simulink model "MatlabNetDDE"  (Simulink 7.3)
settings: Solver=ode3  StartTime=0.0  StopTime=inf  FixedStep=1  RelTol=1e-3
libraries: ddelib x8
settings Model: Creator=Marcin  LastModifiedBy=Marcin  ExtModeBatchMode=on  BufferReuse=off
settings DataIOCC: SaveOutput=off  SaveTime=off
settings OptimizationCC: BlockReduction=off  ConditionallyExecuteInputs=off  OptimizeBlockIOStorage=off  BufferReuse=off  ExpressionFolding=off  EnableMemcpy=off  FoldNonRolledExpr=off  LocalBlockOutputs=off  EfficientMapNaN2IntZero=off
settings RTWCC: GenerateMakefile=off  GenerateReport=on  RetainRTWFile=on  ProcessScript=grt_make_rtw_hook  LaunchReport=on  TargetLang=C++  RTWCompilerOptimization=On
settings CodeAppCC: ForceParamTrailComments=on

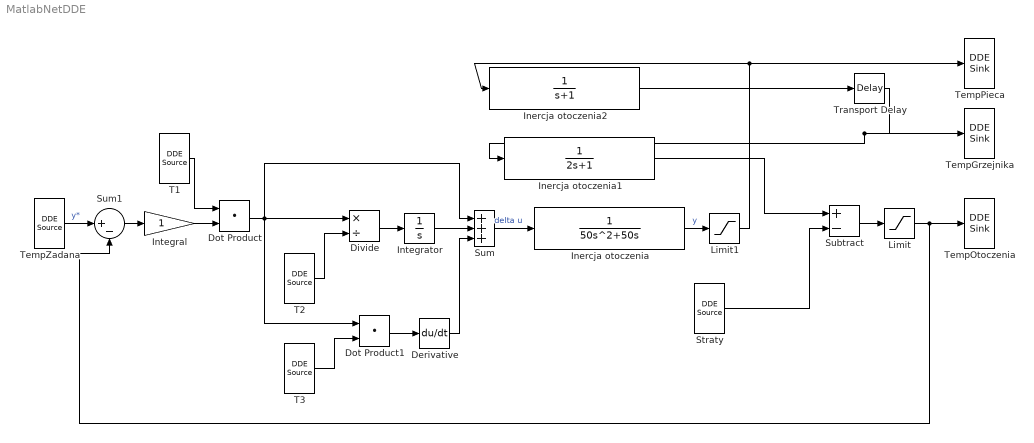
== system MatlabNetDDE ==
  Derivative : Derivative
  Divide : Product  Inputs=*/  OutDataType=fixdt(1, 16)  OutScaling=2^-10
  Dot Product : DotProduct  OutDataType=fixdt(1, 16)  OutScaling=2^-10  InputSameDT=on  OutDataTypeStr=Inherit: Inherit via internal rule
  Dot Product1 : DotProduct  OutDataType=fixdt(1, 16)  OutScaling=2^-10  InputSameDT=on  OutDataTypeStr=Inherit: Inherit via internal rule
  Inercja otoczenia : TransferFcn  Denominator=[50 50 0]
  Inercja otoczenia1 : TransferFcn  Denominator=[2 1]
  Inercja otoczenia2 : TransferFcn  Denominator=[1 1]
  Integral : Gain  ParameterDataType=sfix(16)  ParameterScaling=2^0  OutDataType=sfix(16)  OutScaling=2^0  SaturateOnIntegerOverflow=on  OutDataTypeStr=Inherit: Same as input  ParamDataTypeStr=Inherit: Same as input
  Integrator : Integrator
  Limit : Saturate  UpperLimit=100  LowerLimit=0  OutDataType=fixdt(1, 16)  OutScaling=2^0
  Limit1 : Saturate  UpperLimit=100  LowerLimit=0  OutDataType=fixdt(1, 16)  OutScaling=2^0
  Straty : ddelib/DDE Source  SystemSampleTime=-1  service='\\PC3\NDDE$'  topic='intouch$'  item='Straty'
  Subtract : Sum  Inputs=+-  OutDataType=fixdt(1, 16)  OutScaling=2^-10
  Sum : Sum  Inputs=+++  OutDataType=sfix(16)  OutScaling=2^0  SaturateOnIntegerOverflow=on  InputSameDT=on  OutDataTypeStr=Inherit: Same as first input
  Sum1 : Sum  Inputs=|+-  OutDataType=sfix(16)  OutScaling=2^0  SaturateOnIntegerOverflow=on
  T1 : ddelib/DDE Source  SystemSampleTime=-1  service='\\PC3\NDDE$'  topic='intouch$'  item='T1'
  T2 : ddelib/DDE Source  SystemSampleTime=-1  service='\\PC3\NDDE$'  topic='intouch$'  item='T2'
  T3 : ddelib/DDE Source  SystemSampleTime=-1  service='\\PC3\NDDE$'  topic='intouch$'  item='T3'
  TempGrzejnika : ddelib/DDE Sink  SystemSampleTime=-1  service='\\PC3\NDDE$'  topic='intouch$'  item='TempGrzejnika'
  TempOtoczenia : ddelib/DDE Sink  SystemSampleTime=-1  service='\\PC3\NDDE$'  topic='intouch$'  item='TempOtoczenia'
  TempPieca : ddelib/DDE Sink  SystemSampleTime=-1  service='\\PC3\NDDE$'  topic='intouch$'  item='TempPieca'
  TempZadana : ddelib/DDE Source  SystemSampleTime=-1  service='\\PC3\NDDE$'  topic='intouch$'  item='TempZadanaOtoczenia'
  Transport Delay : TransportDelay
  wires:
  Integrator/1 -> Sum/2
  Sum/1 -> Inercja otoczenia/1  "delta u"
  Divide/1 -> Integrator/1
  Dot Product1/1 -> Derivative/1
  T3/1 -> Dot Product1/2
  T1/1 -> Dot Product/1
  Sum1/1 -> Integral/1
  Dot Product/1 -> Divide/1, Dot Product1/1, Sum/1
  T2/1 -> Divide/2
  Integral/1 -> Dot Product/2
  Derivative/1 -> Sum/3
  TempZadana/1 -> Sum1/1  "y*"
  Limit/1 -> TempOtoczenia/1, Sum1/2
  Subtract/1 -> Limit/1
  Straty/1 -> Subtract/2
  Transport Delay/1 -> TempGrzejnika/1, Inercja otoczenia1/1
  Inercja otoczenia1/1 -> Subtract/1
  Inercja otoczenia2/1 -> Transport Delay/1
  Inercja otoczenia/1 -> Limit1/1  "y"
  Limit1/1 -> TempPieca/1, Inercja otoczenia2/1
